simulink model "EMG_FES2_simulations"  (R2020b)
settings: Solver=FixedStepAuto  StartTime=0.0  StopTime=500  FixedStep=1/Fs  RelTol=1e-3  EnableMultiTasking=on
InitFcn:
  | Fs=1000;%Hz
undefined symbols (not defined in the file or in its folder): fdesignblkfcn, gcbh
libraries: simulink x3, dspswit3 x3, dspinverses x3, dspfdesign x1, dspstat3 x1
settings Model: Creator=bethel.osuagwu  LastModifiedBy=julie
settings DataIOCC: LimitDataPoints=on  SaveFormat=Array  ReturnWorkspaceOutputs=off
settings OptimizationCC: LifeSpan=inf
settings DebuggingCC: SolverPrmCheckMsg=warning  SFUnexpectedBacktrackingDiag=warning  SFNoUnconditionalDefaultTransitionDiag=warning  SFExecutionAtInitializationDiag=none  ArithmeticOperatorsInVariantConditions=warning
settings HardwareCC: ProdBitPerPointer=32  ProdBitPerSizeT=32  ProdBitPerPtrDiffT=32  ProdLargestAtomicFloat=None  ProdIntDivRoundTo=Undefined  ProdEndianess=Unspecified  ProdWordSize=32  ProdHWDeviceType=32-bit Generic
settings ModelReferenceCC: PropagateSignalLabelsOutOfModel=off
settings SFSimCC: SimUseLocalCustomCode=off  CustomCodeUndefinedFunction=UseInterfaceOnly
settings RTWCC: RTWUseLocalCustomCode=off
settings CodeAppCC: StateflowObjectComments=on
settings GRTTargetCC: TargetLangStandard=C89/C90 (ANSI)
settings ConfigComp: CovMetricSettings=dw  CovSaveCumulativeToWorkspaceVar=on  CovSaveSingleToWorkspaceVar=on  CovExternalEMLEnable=off  CovSFcnEnable=off

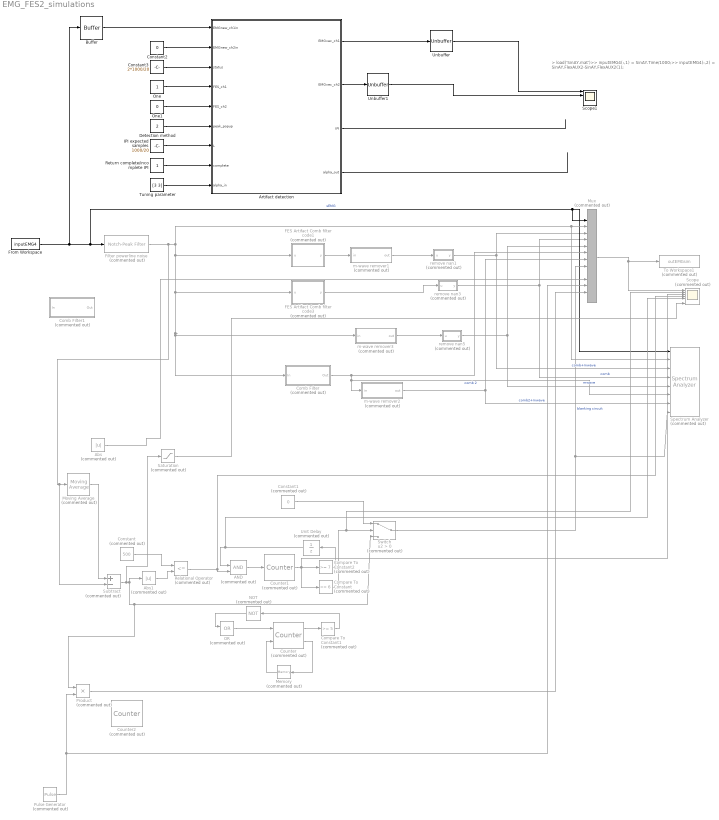
== system EMG_FES2_simulations ==
  note: > load('SinAY.mat')>> inputEMG4(:,1) = SinAY.Time/1000;>> inputEMG4(:,2) = SinAY.FlexAUX2-SinAY.FlexAUX2(1);
  AND : Logic  Commented=on  IconShape=distinctive  AllPortsSameDT=off  OutDataTypeStr=boolean
  Abs : Abs  Commented=on
  Abs1 : Abs  Commented=on
  Artifact detection : MATLAB Function  TreatAsAtomicUnit=on
  Buffer : Buffer  N=2*1000/20  OutputFrames=off
  Comb Filter : Subsystem  Commented=on  DialogController=fdesignblkfcn  InitFcn=fdesignblkfcn(gcbh, {'InitFcn'});  mask(Comb Filter){}
      mask help: Design a Comb Filter
      settings: CopyFcn=fdesignblkfcn(gcbh, {'CopyFcn'});
      mask Help: helpview(mapfilelocation('dsp'), 'dspcombfilter');
      mask Display: disp('Comb');
  Comb Filter1 : Subsystem  Commented=on  DialogController=fdesignblkfcn  InitFcn=fdesignblkfcn(gcbh, {'InitFcn'});  mask(Comb Filter){}
      mask help: Design a Comb Filter
      settings: CopyFcn=fdesignblkfcn(gcbh, {'CopyFcn'});
      mask Help: helpview(mapfilelocation('dsp'), 'dspcombfilter');
      mask Display: disp('Comb');
  Compare To Constant : simulink/Logic and Bit Operations/Compare To Constant  Commented=on  relop=<=  const=6  OutDataTypeStr=boolean
  Compare To Constant1 : simulink/Logic and Bit Operations/Compare To Constant  Commented=on  relop=>=  const=5  OutDataTypeStr=boolean
  Compare To Constant2 : simulink/Logic and Bit Operations/Compare To Constant  Commented=on  relop=>=  const=7  OutDataTypeStr=boolean
  Constant : Constant  Commented=on  Value=500
  Constant1 : Constant  Commented=on  Value=0
  Constant2 : Constant  Value=0
  Constant3 : Constant  Value=2*1000/20
  Counter : dspswit3/Counter  Commented=on  Direction=Up  CountEvent=Non-zero sample  CounterSize=User defined  MaxCount=5  InitialCount=0  Output=Count and Hit  HitValue=5  ResetInput=on  SamplesPerFrame=1  Ts=1  CntDtype=double  HitDtype=Logical
  Counter1 : dspswit3/Counter  Commented=on  Direction=Up  CountEvent=Free running  CounterSize=User defined  MaxCount=1000  InitialCount=0  Output=Count  HitValue=5  ResetInput=on  SamplesPerFrame=1  Ts=-1  CntDtype=double  HitDtype=Logical
  Counter2 : dspswit3/Counter  Commented=on  Direction=Up  CountEvent=Free running  CounterSize=User defined  MaxCount=255  InitialCount=0  Output=Count and Hit  HitValue=50  ResetInput=on  SamplesPerFrame=1  Ts=-1  CntDtype=double  HitDtype=Logical
  Detection method : Constant  Value=2
  FES Artifact Comb filter code1 : MATLAB Function  Commented=on  TreatAsAtomicUnit=on
  FES Artifact Comb filter code3 : MATLAB Function  Commented=on  TreatAsAtomicUnit=on
  Filter powerline noise : dspfdesign/Notch-Peak Filter  Commented=on  Specification=Quality factor and center frequency  BandwidthPort=off  Bandwidth=50  QualityFactorPort=off  QualityFactor=32  CenterFrequencyPort=off  CenterFrequency=50  BandwidthCoefficientPort=off  BandwidthCoefficient=0.72654  CenterFrequencyCoefficientPort=off  CenterFrequencyCoefficient=0  Output=Notch  InheritSampleRate=off  SampleRate=1000  SimulateUsing=Code generation
      settings: SourceProductBaseCode=DS
  From Workspace : FromWorkspace  VariableName=inputEMG4  SampleTime=1/Fs  OutputAfterFinalValue=Setting to zero
  IPI expected samples : Constant  Value=1000/20
  Memory : Memory  Commented=on
  Moving Average : dspstat3/Moving Average  Commented=on  Method=Sliding window  ForgettingFactorPort=off  SpecifyWindowLength=on  WindowLength=2000  ForgettingFactor=0.9  SimulateUsing=Code generation
  Mux : Mux  Commented=on  Inputs=12
  NOT : Logic  Commented=on  Operator=NOT  IconShape=distinctive  AllPortsSameDT=off  OutDataTypeStr=boolean
  OR : Logic  Commented=on  Operator=OR  IconShape=distinctive  AllPortsSameDT=off  OutDataTypeStr=boolean
  One : Constant  OutDataTypeStr=Inherit: Inherit via back propagation
  One1 : Constant  Value=0  OutDataTypeStr=Inherit: Inherit via back propagation
  Product : Product  Commented=on
  Pulse Generator : DiscretePulseGenerator  Commented=on  Period=50  PulseWidth=40  PhaseDelay=10  SampleTime=-1
  Relational Operator : RelationalOperator  Commented=on  Operator=<=  OutDataTypeStr=boolean  RndMeth=Simplest
  Return complete/incomplete IPI : Constant
  Saturation : Saturate  Commented=on  UpperLimit=250  LowerLimit=-250
  Scope : Scope  Commented=on  NumInputPorts=7
  Scope1 : Scope  NumInputPorts=4
  Spectrum Analyzer : SpectrumAnalyzer  Commented=on  NumInputPorts=8
  Subtract : Sum  Commented=on  Inputs=+-
  Switch : Switch  Commented=on  Criteria=u2 > Threshold
  To Workspace1 : ToWorkspace  Commented=on  VariableName=outEMGsim  SampleTime=-1
  Tuning parameter : Constant  Value=[3 3]
  Unbuffer : Unbuffer
  Unbuffer1 : Unbuffer
  Unit Delay : UnitDelay  Commented=on  SampleTime=-1  HasFrameUpgradeWarning=on
  m-wave remover1 : Subsystem  Commented=on
  m-wave remover2 : Subsystem  Commented=on
  m-wave remover3 : Subsystem  Commented=on
  remove nan1 : MATLAB Function  Commented=on  TreatAsAtomicUnit=on
  remove nan3 : MATLAB Function  Commented=on  TreatAsAtomicUnit=on
  remove nan5 : MATLAB Function  Commented=on  TreatAsAtomicUnit=on
  wires:
  Mux/1 -> To Workspace1/1, Scope/1
  m-wave remover3/1(out) -> remove nan5/1(u)
  FES Artifact Comb filter code3/1(y) -> remove nan3/1(u)
  m-wave remover1/1(out) -> remove nan1/1(u)
  FES Artifact Comb filter code1/1(y) -> m-wave remover1/1(in)
  remove nan1/1(y) -> Spectrum Analyzer/3, Mux/3  "comb+mwave"
  remove nan3/1(y) -> Spectrum Analyzer/4, Mux/4  "comb"
  remove nan5/1(y) -> Spectrum Analyzer/5, Mux/5  "mwave"
  From Workspace/1 -> Buffer/1, Filter powerline noise/1, Spectrum Analyzer/1, Mux/1  "sEMG"
  Filter powerline noise/1 -> Subtract/2, Moving Average/1, FES Artifact Comb filter code1/1(u), FES Artifact Comb filter code3/1(u), m-wave remover3/1(in), Comb Filter/1(In), Mux/2, Spectrum Analyzer/2
  Comb Filter/1(Out) -> m-wave remover2/1(in), Spectrum Analyzer/6, Mux/6  "comb 2"
  m-wave remover2/1(out) -> Spectrum Analyzer/7, Mux/7  "comb2+mwave"
  Switch/1 -> Spectrum Analyzer/8, Mux/8  "blanking circuit"
  Abs/1 -> Mux/10
  Moving Average/1 -> Subtract/1
  Constant/1 -> Relational Operator/1
  Subtract/1 -> Saturation/1, Abs1/1, Product/1, Switch/3
  Constant1/1 -> Switch/1
  Relational Operator/1 -> Scope/4, AND/2
  Memory/1 -> Counter/2
  NOT/1 -> OR/1
  OR/1 -> Counter/1
  Counter/2 -> Memory/1
  Compare To Constant1/1 -> NOT/1
  Counter/1 -> Compare To Constant1/1
  AND/1 -> Counter1/1
  Counter1/1 -> Compare To Constant/1, Scope/3, Compare To Constant2/1
  Compare To Constant/1 -> Scope/2, Switch/2
  Unit Delay/1 -> Scope/5, AND/1
  Compare To Constant2/1 -> Unit Delay/1
  Abs1/1 -> Relational Operator/2
  Saturation/1 -> Scope/7
  Pulse Generator/1 -> Mux/11, Product/2
  Product/1 -> Mux/12
  Detection method/1 -> Artifact detection/6(peak_popup)
  Tuning parameter/1 -> Artifact detection/9(alpha_in)
  IPI expected samples/1 -> Artifact detection/7(L)
  Return complete/incomplete IPI/1 -> Artifact detection/8(complete)
  One/1 -> Artifact detection/4(FES_ch1)
  One1/1 -> Artifact detection/5(FES_ch2)
  Constant2/1 -> Artifact detection/2(EMGnew_ch2in)
  Buffer/1 -> Artifact detection/1(EMGnew_ch1in)
  Constant3/1 -> Artifact detection/3(status)
  Artifact detection/2(EMGvec_ch2) -> Unbuffer1/1
  Artifact detection/1(EMGvec_ch1) -> Unbuffer/1
  Unbuffer/1 -> Scope1/1
  Unbuffer1/1 -> Scope1/2
  Artifact detection/3(IPI) -> ?
  Artifact detection/4(alpha_out) -> ?

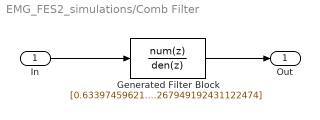
== system EMG_FES2_simulations/Comb Filter ==
  In : Inport
  Generated Filter Block : DiscreteFilter  Tag=BlockMethodSubSystem  Numerator=[0.633974596215561292 0 0 0 0 0 0 0 0 0 0 0 0 0 0 0 0 0 0 0 0 0 0 0 0 0 0 0 0 0 0 0 0 0 0 0 0 0 0 0 0 0 0 0 0 0 0 0 0 0 -0.633974596215561292]  Denominator=[1 0 0 0 0 0 0 0 0 0 0 0 0 0 0 0 0 0 0 0 0 0 0 0 0 0 0 0 0 0 0 0 0 0 0 0 0 0 0 0 0 0 0 0 0 0 0 0 0 0 -0.267949192431122474]  InputProcessing=Columns as channels (frame based)  FilterStructure=Direct form II transposed  a0EqualsOne=on
  Out : Outport  VectorParamsAs1DForOutWhenUnconnected=off
  wires:
  Generated Filter Block/1 -> Out/1
  In/1 -> Generated Filter Block/1

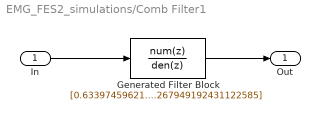
== system EMG_FES2_simulations/Comb Filter1 ==
  In : Inport
  Generated Filter Block : DiscreteFilter  Tag=BlockMethodSubSystem  Numerator=[0.633974596215561292 0 0 0 0 0 0 0 0 0 0 0 0 0 0 0 0 0 0 0 -0.633974596215561292]  Denominator=[1 0 0 0 0 0 0 0 0 0 0 0 0 0 0 0 0 0 0 0 -0.267949192431122585]  InputProcessing=Columns as channels (frame based)  a0EqualsOne=on
  Out : Outport  VectorParamsAs1DForOutWhenUnconnected=off
  wires:
  Generated Filter Block/1 -> Out/1
  In/1 -> Generated Filter Block/1

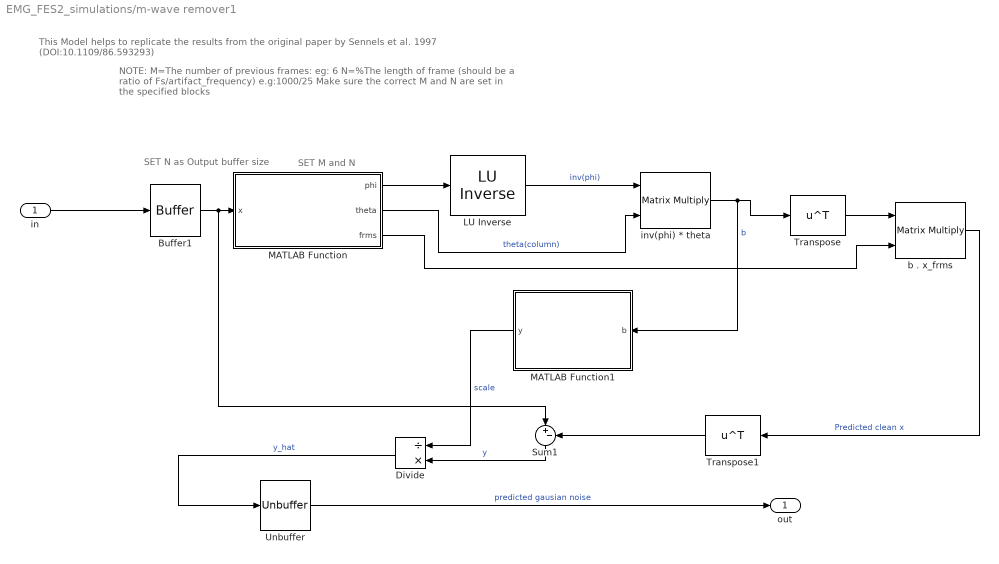
== system EMG_FES2_simulations/m-wave remover1 ==
  note: This Model helps to replicate the results from the original paper by Sennels et al. 1997 (DOI:10.1109/86.593293)
  note: SET M and N
  note: SET N as Output
      | buffer size
  note: NOTE:
      | M=The number of previous frames: eg: 6
      | N=%The length of frame (should be a ratio of Fs/artifact_frequency) e.g:1000/25
      | Make sure the correct M and N are set in the specified blocks
  in : Inport
  " LU Inverse" : dspinverses/ LU Inverse
  Buffer1 : Buffer  N=1000/20
  Divide : Product  Inputs=/*
  MATLAB Function : MATLAB Function  TreatAsAtomicUnit=on
  MATLAB Function1 : MATLAB Function  TreatAsAtomicUnit=on
  Sum1 : Sum  Inputs=|+-
  Transpose : Math  Operator=transpose  SaturateOnIntegerOverflow=on
  Transpose1 : Math  Operator=transpose  SaturateOnIntegerOverflow=on
  Unbuffer : Unbuffer
  b . x_frms : Product  Multiplication=Matrix(*)
  inv(phi) * theta : Product  Multiplication=Matrix(*)
  out : Outport
  wires:
  in/1 -> Buffer1/1
  Divide/1 -> Unbuffer/1  "y_hat"
  MATLAB Function1/1(y) -> Divide/1  "scale"
  Sum1/1 -> Divide/2  "y"
  Transpose1/1 -> Sum1/2
  b . x_frms/1 -> Transpose1/1  "Predicted clean x"
  Transpose/1 -> b . x_frms/1
  MATLAB Function/3(frms) -> b . x_frms/2
  Unbuffer/1 -> out/1  "predicted gausian noise"
  inv(phi) * theta/1 -> Transpose/1, MATLAB Function1/1(b)  "b"
  " LU Inverse"/1 -> inv(phi) * theta/1  "inv(phi)"
  MATLAB Function/2(theta) -> inv(phi) * theta/2  "theta(column)"
  MATLAB Function/1(phi) -> " LU Inverse"/1
  Buffer1/1 -> MATLAB Function/1(x), Sum1/1

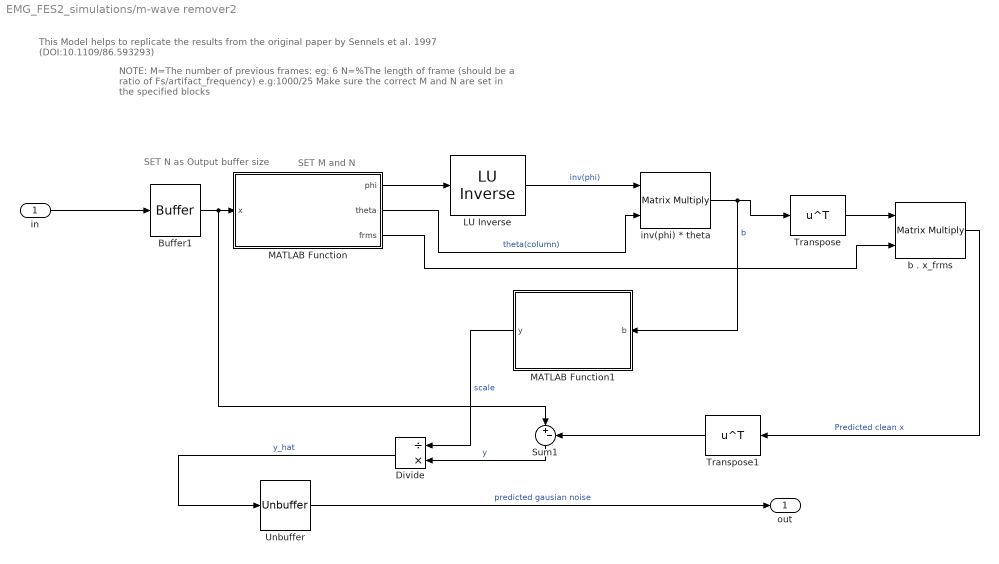
== system EMG_FES2_simulations/m-wave remover2 ==
  note: This Model helps to replicate the results from the original paper by Sennels et al. 1997 (DOI:10.1109/86.593293)
  note: SET M and N
  note: SET N as Output
      | buffer size
  note: NOTE:
      | M=The number of previous frames: eg: 6
      | N=%The length of frame (should be a ratio of Fs/artifact_frequency) e.g:1000/25
      | Make sure the correct M and N are set in the specified blocks
  in : Inport
  " LU Inverse" : dspinverses/ LU Inverse
  Buffer1 : Buffer  N=1000/20
  Divide : Product  Inputs=/*
  MATLAB Function : MATLAB Function  TreatAsAtomicUnit=on
  MATLAB Function1 : MATLAB Function  TreatAsAtomicUnit=on
  Sum1 : Sum  Inputs=|+-
  Transpose : Math  Operator=transpose  SaturateOnIntegerOverflow=on
  Transpose1 : Math  Operator=transpose  SaturateOnIntegerOverflow=on
  Unbuffer : Unbuffer
  b . x_frms : Product  Multiplication=Matrix(*)
  inv(phi) * theta : Product  Multiplication=Matrix(*)
  out : Outport
  wires:
  in/1 -> Buffer1/1
  Divide/1 -> Unbuffer/1  "y_hat"
  MATLAB Function1/1(y) -> Divide/1  "scale"
  Sum1/1 -> Divide/2  "y"
  Transpose1/1 -> Sum1/2
  b . x_frms/1 -> Transpose1/1  "Predicted clean x"
  Transpose/1 -> b . x_frms/1
  MATLAB Function/3(frms) -> b . x_frms/2
  Unbuffer/1 -> out/1  "predicted gausian noise"
  inv(phi) * theta/1 -> Transpose/1, MATLAB Function1/1(b)  "b"
  " LU Inverse"/1 -> inv(phi) * theta/1  "inv(phi)"
  MATLAB Function/2(theta) -> inv(phi) * theta/2  "theta(column)"
  MATLAB Function/1(phi) -> " LU Inverse"/1
  Buffer1/1 -> MATLAB Function/1(x), Sum1/1

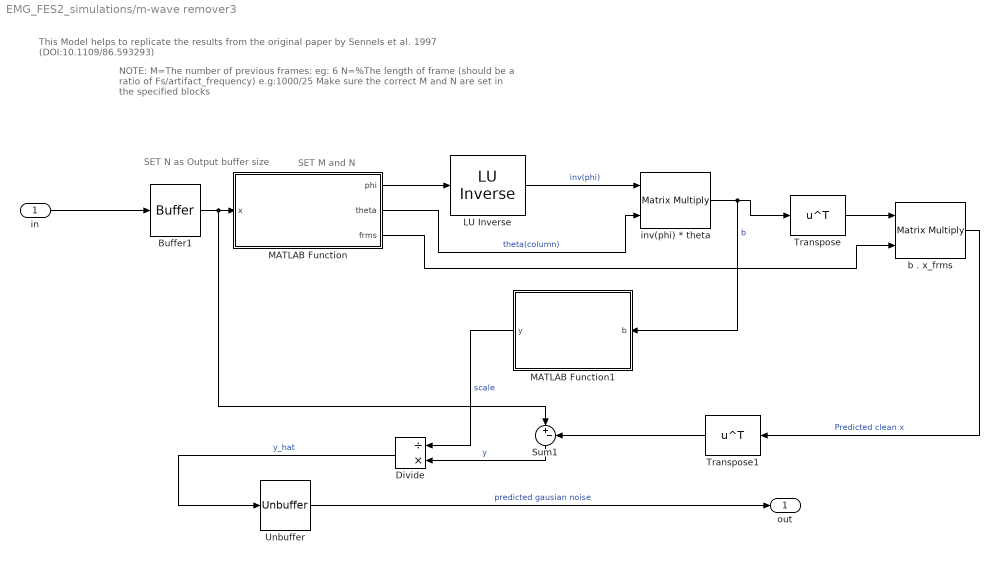
== system EMG_FES2_simulations/m-wave remover3 ==
  note: This Model helps to replicate the results from the original paper by Sennels et al. 1997 (DOI:10.1109/86.593293)
  note: SET M and N
  note: SET N as Output
      | buffer size
  note: NOTE:
      | M=The number of previous frames: eg: 6
      | N=%The length of frame (should be a ratio of Fs/artifact_frequency) e.g:1000/25
      | Make sure the correct M and N are set in the specified blocks
  in : Inport
  " LU Inverse" : dspinverses/ LU Inverse
  Buffer1 : Buffer  N=1000/20
  Divide : Product  Inputs=/*
  MATLAB Function : MATLAB Function  TreatAsAtomicUnit=on
  MATLAB Function1 : MATLAB Function  TreatAsAtomicUnit=on
  Sum1 : Sum  Inputs=|+-
  Transpose : Math  Operator=transpose  SaturateOnIntegerOverflow=on
  Transpose1 : Math  Operator=transpose  SaturateOnIntegerOverflow=on
  Unbuffer : Unbuffer
  b . x_frms : Product  Multiplication=Matrix(*)
  inv(phi) * theta : Product  Multiplication=Matrix(*)
  out : Outport
  wires:
  in/1 -> Buffer1/1
  Divide/1 -> Unbuffer/1  "y_hat"
  MATLAB Function1/1(y) -> Divide/1  "scale"
  Sum1/1 -> Divide/2  "y"
  Transpose1/1 -> Sum1/2
  b . x_frms/1 -> Transpose1/1  "Predicted clean x"
  Transpose/1 -> b . x_frms/1
  MATLAB Function/3(frms) -> b . x_frms/2
  Unbuffer/1 -> out/1  "predicted gausian noise"
  inv(phi) * theta/1 -> Transpose/1, MATLAB Function1/1(b)  "b"
  " LU Inverse"/1 -> inv(phi) * theta/1  "inv(phi)"
  MATLAB Function/2(theta) -> inv(phi) * theta/2  "theta(column)"
  MATLAB Function/1(phi) -> " LU Inverse"/1
  Buffer1/1 -> MATLAB Function/1(x), Sum1/1

== matlab function EMG_FES2_simulations/FES Artifact Comb filter code1 ==
  data: u input; y output
function y  = fcn(u)
%#codegen

persistent u_mem;
fes_freq=20;%FES frequency
Fs=1000;%EMG/data samplerate
K=round(Fs/fes_freq); %Comb filter order = (1/fes_freq)*Fs
a=-1;%{-1 to 0}
if isempty(u_mem)
    u_mem=zeros(K,1);
end





%% Comb filtering
% Forward comb
y=u+ a*u_mem(1);



u_mem(1:end-1)=u_mem(2:end);
u_mem(end)=u;
end





%

== matlab function EMG_FES2_simulations/FES Artifact Comb filter code3 ==
  data: u input; y output
function y  = fcn(u)
%#codegen

persistent u_mem;
fes_freq=20;%FES frequency
Fs=1000;%EMG/data samplerate
K=round(Fs/fes_freq); %Comb filter order = (1/fes_freq)*Fs
a=-1;%{-1 to 0}
if isempty(u_mem)
    u_mem=zeros(K,1);
end





%% Comb filtering
% Forward comb
y=u+ a*u_mem(1);



u_mem(1:end-1)=u_mem(2:end);
u_mem(end)=u;
end





%

== matlab function EMG_FES2_simulations/m-wave remover2/MATLAB Function ==
  data: x input; phi output double; theta output; frms output
function [phi,theta,frms] = fcn(x)
%#codegen
persistent t_sample phi_mem  frms_mem ;

%General param
M=6; %The number of previous frames 
N=1000/20; %The length of frame (should be a ratio of Fs/artifact_frequency)

% Performance parameter
freshPhi =1;% when =1:recompute phi(covariance matix) all the phi; when =0:update phi with only new values

if isempty(t_sample)
    t_sample=0;
    frms_mem=zeros(M,N);
    
    phi_mem=zeros(M,M);
end
t_sample=t_sample+1;

%make x a row vector
x=x';


%% compute phi
frms=frms_mem;
%equ 7 and 8
if(freshPhi)
    % compute phi fresh all the time
    phi=(frms*frms');
else
    %we can compute only the required column (first) and row (first)of phi
    %matrix and push the new values into phi
    phi_mem(2:end,2:end)=phi_mem(1:end-1,1:end-1);
    phi_mem(1,:)=frms(1,:)*frms';
    phi_mem(:,1)=phi_mem(1,:)';
    %phi-phi_mem
    phi=phi_mem;
end


%% compute theta
theta=(x*frms')';
%t_sample
%if t_sample==15
%    y=4;
%end


%% update frame
frms_mem(2:end,:)=frms_mem(1:end-1,:);
frms_mem(1,:)=x;

== matlab function EMG_FES2_simulations/remove nan1 ==
  data: u input; y output
function y  = fcn(u)
%#codegen

y=u;
if isnan(y)
    y=0;
end





%

== matlab function EMG_FES2_simulations/m-wave remover2/MATLAB Function1 ==
  data: b input; y output
function y = fcn(b)
%#codegen


y = sqrt(1+sum(b.^2));
%       OR
%y = (1+sum(b));%approximated for speed

== matlab function EMG_FES2_simulations/remove nan3 ==
  data: u input; y output
function y  = fcn(u)
%#codegen

y=u;
if isnan(y)
    y=0;
end





%

== matlab function EMG_FES2_simulations/Artifact detection ==
  data: EMGnew_ch1in input; EMGvec_ch1 output; EMGnew_ch2in input; status input; FES_ch1 input; FES_ch2 input; peak_popup input; L input; complete input; alpha_in input; EMGvec_ch2 output; IPI output; alpha_out output
%% %%%%%%%%%%%%%%%%%%%%%%%%%%%%%%%%%%%%%%%%%%%%%%%%%%%%%%%%%%%%%%%%%%%%%%%%
% block artifactDetection
% by Ana de Sousa (anacsousa@lara.unb.br)
% Last update: Feb-2018
%% %%%%%%%%%%%%%%%%%%%%%%%%%%%%%%%%%%%%%%%%%%%%%%%%%%%%%%%%%%%%%%%%%%%%%%%%

function [EMGvec_ch1, EMGvec_ch2, IPI, alpha_out]   = artifactDetection(EMGnew_ch1in, EMGnew_ch2in, status, FES_ch1, FES_ch2, peak_popup, L, complete, alpha_in)

    %% transpose if not column
    if isrow(EMGnew_ch1in)
        EMGnew_ch1 = EMGnew_ch1in';
    else
        EMGnew_ch1 = EMGnew_ch1in;
    end    
    if isrow(EMGnew_ch2in)
        EMGnew_ch2 = EMGnew_ch2in';
    else
        EMGnew_ch2 = EMGnew_ch2in;
    end

    %% Definition of parameters  
    b = 3.1;
    buffer_size = ceil(L*b);
    buffer_offsets_size = 5;
    n_stims = floor(b)+1;   
    ch_conn = [0,0];
    
    %% Step 0: pre-check (Verification of connected channels)
    if EMGnew_ch1 == 0
        ch_conn(1) = 0;
    else
        ch_conn(1) = 1;
    end
    
    if EMGnew_ch2 == 0
        ch_conn(2) = 0;
    else
        ch_conn(2) = 1;
    end
    
    %% Step 1: create and update buffers
    persistent  emg_buffer; 
    if isempty(emg_buffer)
        emg_buffer = bound_buffer2(buffer_size);
    end
    
    persistent  buffer_offsets_ch1;
    if isempty(buffer_offsets_ch1) 
        buffer_offsets_ch1 = bound_buffer(buffer_offsets_size);
    end
    
    persistent  buffer_offsets_ch2;
    if isempty(buffer_offsets_ch2) 
        buffer_offsets_ch2 = bound_buffer(buffer_offsets_size);
    end
    
    persistent  last_stim; 
    if isempty(last_stim)
        last_stim = bound_stim(n_stims);
    end
    
    %% alpha definitions
    persistent  alpha;
    if isempty(alpha) 
        alpha = alpha_in(2); % init alpha with second value
    end
    
    % Updates buffer from EMG data
    EMGstatus = int16(status(1));
    
    if (EMGstatus >= 1)   % ch1
        if EMGstatus > buffer_size % limit EMGstatus size to avoid errors if incorrect freq is put
            EMGstatus = int16(buffer_size);
            disp('Warning: status > buffer size, check EMG and stimulation frequencies.');
        end
        if size(EMGnew_ch1,1) > 1
            emg_buffer(1:buffer_size,1) = [emg_buffer(EMGstatus+1:buffer_size,1);EMGnew_ch1(1:EMGstatus)];
        end
    end
    
    if (EMGstatus >= 1)   % ch2
        if size(EMGnew_ch2,1) > 1
            emg_buffer(1:buffer_size,2) = [emg_buffer(EMGstatus+1:buffer_size,2);EMGnew_ch2(1:EMGstatus)];
        end
    end
    
    % Updates buffer from FES data
    stim = or(FES_ch1(1),FES_ch2(1));    
    last_stim(1:n_stims) = [last_stim(2:n_stims);stim];
    idx = last_stim ~= 0; 
    n_stims = sum(idx(:)); % # of artifacts expected, relates to buff_size;
        
    %% Step 2: artifacts detection (all artifacts found)
    IPI_c = buffer_size - L;
    IPI_i = buffer_size - L;
    
    % considers if channels are conn and stimulated 
    if (ch_conn(1)==1)||(ch_conn(2)==1) 
        if n_stims % if there is any pulse
            
            if (~isequal(last_stim,[0;0;0;1]))&&(~isequal(last_stim,[1;0;0;0])) % transitions of stim
                % find all points
                [all_pts] = choose_algorithm(peak_popup,alpha,emg_buffer);
                
                    %% consider # clusters vs alpha 
                    n_clusters = count_clusters(all_pts,L);
                    
                    %% if automatic alpha was chosen:
                    if alpha_in(1)
                        n_exp_pulses = 3;                        
                        d_alpha = n_clusters - n_exp_pulses;
                        
                        % if found pulses are different from expected pulses
                        if ~((n_clusters == 3) || (n_clusters == 4) || (n_clusters == 5))
                            % alpha limits
                            switch peak_popup
                                case 1 % 'var'
                                    ss = 0.1;
                                    alpha = alpha*(1+sign(d_alpha)*ss);
                                    
                                    if alpha < 10^-3
                                        alpha = 10^-3;
                                    elseif alpha > 5
                                        alpha = 5;
                                    end
                                    
                                case 2 % 'MAD'  
                                    ss = 0.1;
                                    alpha = alpha*(1+sign(d_alpha)*ss);
                                    
                                    if alpha < 2
                                        alpha = 2;
                                    elseif alpha > 5000
                                        alpha = 5000;
                                    end
                                case 3 % 'q'   
                                    ss = 0.01;
                                    alpha = alpha*(1+sign(d_alpha)*ss);
                                    
                                    if alpha < 0.9 %% simulink does not understand that we already bounded it...
                                        alpha = 0.9;
                                    elseif alpha >  0.985
                                        alpha = 0.985;
                                    end
                                otherwise % 'otherwise'
                                    error('No algorithm was selected.');
                            end   
                        end
                    end

                %% Step 3: determine IPI based on found artifacts
                [IPI_c,IPI_i] = cluster_peaks(all_pts, L, last_stim, n_stims);
            end
        end
    end
    
    %% Step 4: extract last full emg period
    if complete % return IPI complete or incomplete
        IPI = IPI_c;        
        % check if enough samples  
        if (IPI(1) < 0 )||(IPI(1) > buffer_size - L) 
            IPI(1) = buffer_size - L;
        end
    else
        IPI = IPI_i;
    end
    
    [ EMGvec_ch1, buffer_offsets_ch1 ] = extractLastFullEMG(IPI, emg_buffer(:,1), buffer_offsets_ch1, L, complete); 
    [ EMGvec_ch2, buffer_offsets_ch2 ] = extractLastFullEMG(IPI, emg_buffer(:,2), buffer_offsets_ch2, L, complete);
    
    alpha_out = alpha;
end

%% %%%%%%%%%%%%%%%%%%%%%%%%%%%%%%%%%%%%%%%%%%%%%%%%%%%%%%%%%%%%%%%%%%%%%%%%%
%% %%%%%%%%%%%%%%%%%%%%%%%%%%%%%%%%%%%%%%%%%%%%%%%%%%%%%%%%%%%%%%%%%%%%%%%%%
%% %%%%%%%%%%%%%%%%%%%%%%%%%%%%%%%%%%%%%%%%%%%%%%%%%%%%%%%%%%%%%%%%%%%%%%%%%

%% Specify Upper Bounds for Local Variables
% see more: (https://de.mathworks.com/help/simulink/ug/variable-size-data-when-dynamic-memory-allocation-is-disabled.html)
function y = bound_buffer(n)
    assert(n <= 5*4000/10, 'Buffer size is higher than 2000.'); 
    y = zeros(n,1);
end

function y = bound_buffer2(n)
    assert(n <= 5*4000/10, 'Buffer size is higher than 2000.');
    y = zeros(n,2);
end

function y = bound_stim(n)
    assert(n <= 10, 'Number of stims is higher than 10. '); 
    y = zeros(n,1);
end

function y = bound_vec(n)
    assert(n <= 5*4000/10, 'Buffer size is higher than 2000.'); 
    y = zeros(1,n);
end

%% Choose the algorithm to find all peaks %%%%%%%%%%%%%%%%%%%%%%%%%%%%%%%%%
function [all_IPI] = choose_algorithm(peak_popup,alpha,emg_vec)
    n_loc_found = length(emg_vec);
    all_IPI = zeros(1,n_loc_found);
    
    switch peak_popup
        case 1 % 'std'            
            DE1 = (diff(diff(emg_vec(:,1))));
            DE2 = (diff(diff(emg_vec(:,2))));
            mean_d1 = mean(DE1,'omitnan');  mean_d2 = mean(DE2,'omitnan');
            std_d1 = std(DE1,'omitnan');    std_d2 = std(DE2,'omitnan');
            
            % look for points
            k_max1 = mean_d1+std_d1*alpha;  k_max2 = mean_d2+std_d2*alpha;
            k_min1 = mean_d1-std_d1*alpha;  k_min2 = mean_d2-std_d2*alpha;
            
            loc_found1 = find(DE1 > k_max1 | DE1 < k_min1); %find std1
            loc_found2 = find(DE2 > k_max2 | DE2 < k_min2); %find std2
            loc_found = union(loc_found1,loc_found2);

        case 2 % 'MAD'
            DE1 = (diff(diff(emg_vec(:,1))));
            DE2 = (diff(diff(emg_vec(:,2))));
            mean_d1 = median(DE1,'omitnan');  mean_d2 = median(DE2,'omitnan');
            mad_d1 = mad(DE1,1);            mad_d2 = mad(DE2,1);
            
            % look for points
            k_max1 = mean_d1+mad_d1*alpha;  k_max2 = mean_d2+mad_d2*alpha;
            k_min1 = mean_d1-mad_d1*alpha;  k_min2 = mean_d2-mad_d2*alpha;
            
            loc_found1 = find(DE1 > k_max1 | DE1 < k_min1); %find std1
            loc_found2 = find(DE2 > k_max2 | DE2 < k_min2); %find std2
            loc_found = union(loc_found1,loc_found2);
            
        case 3 % 'quantiles'
            DE1 = (diff(diff(emg_vec(:,1))));
            DE2 = (diff(diff(emg_vec(:,2))));
            
            
            if alpha < 0.9 %% simulink does not understand that we already bounded it...
                alpha = 0.9;
            elseif alpha >  0.985
                alpha = 0.985;
            end

            q_max1 = quantile(DE1,alpha);
            q_min1 = quantile(DE1,1-alpha);
            q_max2 = quantile(DE2,alpha); 
            q_min2 = quantile(DE2,1-alpha);
            loc_found1 = find( DE1>q_max1(1) | DE1<q_min1(1)) ; %find quantiles DE1
            loc_found2 = find( DE2>q_max2(1) | DE2<q_min2(1)) ; %find quantiles DE2
            loc_found = union(loc_found1,loc_found2);   
            
        otherwise % 'otherwise'
            error('No algorithm was selected.');
    end
    
    % Adjust vector to return
    if ~isempty(loc_found)
        a = min(n_loc_found,length(loc_found));  %check which is smaller

        for i=1:a % do not extrapolate the vector
            all_IPI(i) = loc_found(i);
        end
    end  
end

%% Extract last full emg period from last IPI %%%%%%%%%%%%%%%%%%%%%%%%%%%%%
function [ EMGvec, offsets_buffer ] = extractLastFullEMG(IPI, emg_buffer, offsets_buffer, L, complete)

	% Parameters
%     EMGvec = NaN(1,200);
    EMGvec = NaN(1,100);
    buffer_size = length(emg_buffer);
    buffer_size_offsets = length(offsets_buffer); 
    
    %% update the emg vec with the new COMPLETE peak (until L)
    
    %% if IPI is not zero, we return position based on IPI (complete or incomplete)
    if IPI(1) ~= 0
        %% now we consider if it is complete or incomplete
        if complete %% complete
            for i = 1:L 
                EMGvec(i) = emg_buffer(IPI + i);
            end
        else %% incomplete
            %% if there is enough samples, just fill (buffer_size-L)
            if IPI(1) <= buffer_size - L
                for i = 1:L 
                    EMGvec(i) = emg_buffer(IPI + i);
                end
            %% if there is not, fill until possible (buffer_size-IPI)
            else
                for i = 1:buffer_size-IPI 
                    EMGvec(i) = emg_buffer(IPI + i);
                end
            end
        end
    %% otherwise, something went wrong before, so return EMGvec as zero
    else
        for i = 1:L 
            EMGvec(i) = 0;
        end
    end
        
    %% Remove offset
    for i = 1:buffer_size_offsets-1
        offsets_buffer(end-i+1) = offsets_buffer(end-i);
    end
    x = 0;
    c = buffer_size_offsets;
    for i = 1:buffer_size_offsets
        x = x + emg_buffer(ceil(0.8*L) + i);
    end
    offsets_buffer(1) = x/c; %mean

    EMGvec = EMGvec - mean(offsets_buffer);
    EMGvec = EMGvec.'; % return
end


%% Cluster peaks %%%%%%%%%%%%%%%%%%%%%%%%%%%%%%%%%%%%%%%%%%%%%%%%%%%%%%%%%%%
function [IPI_c,IPI_i] = cluster_peaks(all_pts, L, last_stim, n_stims)

    %% parameters
    buffer_size = length(all_pts);
    if ~(last_stim(end) == 0) %adjust # of expected stims
        n_stims = n_stims-1;
    end
    
    %% find clusters and count # of elements in each cluster
    ind_del = all_pts == 0;    points = all_pts;
    points(ind_del) = [];
    changes = find((diff(points) > L*0.1))+1; % find where cluster change
    n_clusters = length(changes) + 1; % # of clusters found
    
    a = zeros(1,n_clusters);
    b = zeros(1,n_clusters);
    
    if(n_clusters > 1) % more than one cluster found
        u = [changes(1)-1, diff(changes), length(points) - changes(end) + 1];        
        % saving first (a) and last (b) points of each cluster (i)
        for i=1:n_clusters
            if i == 1
                a(i) = points(1);
                b(i) = points(changes(i)-1);
            elseif i == n_clusters
                a(i) = points(changes(i-1));
                b(i) = points(end);
            else
                a(i) = points(changes(i-1));
                b(i) = points(changes(i)-1);
            end
        end
    else % only one (or none) cluster found
        u = length(points);
        if ~isempty(points)
            a = points(1);
            b = points(end);
        else
            a = 1;
            b = 1;
        end
    end
        
    %% create base and real vectors
    vec_base = bound_vec(buffer_size);    
    vec_real = bound_vec(buffer_size);
    
    if floor(mean(u)) % base
        if mean(b-a)+1 < ceil(L/2) % limit number of points
            n_pts = ceil(mean(b-a)+1);
        else
            n_pts = ceil(L/2);
        end
    else 
        n_pts = 5;
    end
    
    init = 1;    
    for i = 1:n_stims %vec_base
        vec_base((init + (i-1)*L):init + n_pts + (i-1)*L - 1) = 1;
    end
    
    for i = 1:length(a) %vec_real
        vec_real(a(i)) = 1;
        for j = 1:b(i)-a(i)
            vec_real(a(i)+j) = 1;
        end
    end
    
    %% Correlate vec_base and vec_real to shift them
    [acor,lag] = xcorr(vec_base', vec_real');
    [~,I] = max(abs(acor));
    lagDiff = abs(lag(I));
            
    %% Transition state (#stims = 1), IPI = lagDiff
    % Everthing bellow considers the transitions between on and off stim:
    %   . When the charge shifts on -> off, or off -> on, the stimulator
    %   needs a period to respond in real time.
    %   . Also we need to consider if we want a complete or an incomplete
    %   IPI.
    IPI_c = buffer_size - L;
    IPI_i = buffer_size - L;
    
    % TRANSITIONS
    adjust_diff = 0;
    if isequal(last_stim,[0;0;1;1]) % transition off->on (for IPI_i)
        IPI_i = lagDiff+adjust_diff;
        IPI_c = 0;
    elseif isequal(last_stim,[1;1;0;0]) % transition on->off (for IPI_c)
        new_pos = find( points > 0.95*(lagDiff+L+adjust_diff) ); % look for the 1st pulse after
        if new_pos
            IPI_c = points(new_pos(1))+adjust_diff;
        end
    elseif isequal(last_stim,[0;1;1;1]) % transition off->on (for in and complete)
        IPI_c = lagDiff+2;
        new_pos = find( points > 0.95*(lagDiff+L+adjust_diff) ); % look for next pulse
        if new_pos
            IPI_i = points(new_pos(1))+adjust_diff;
        end
    % STABLE
    else  
        new_pos = find( points > 0.95*(lagDiff+L+adjust_diff) ); % look for the 1st pulse after
        if new_pos
            IPI_c = points(new_pos(1))+adjust_diff;
        end

        new_pos2 = find( points > 0.95*(lagDiff+2*L+adjust_diff) ); % look for the 2nd pulse after
        if new_pos2
            IPI_i = points(new_pos2(1))+adjust_diff;
        end
    end
end

%% Count number of clusters %%%%%%%%%%%%%%%%%%%%%%%%%%%%%%%%%%%%%%%%%%%%%%%%
function n_clusters = count_clusters(all_pts,L)
    % make a vector without the zeros
    ind_del = all_pts == 0;     points = all_pts;
    points(ind_del) = [];  
    
    % count clusters considering a min diff between points
    changes = find((diff(points) > L*0.1))+1;
    n_clusters = length(changes) + 1;
end

== matlab function EMG_FES2_simulations/remove nan5 ==
  data: u input; y output
function y  = fcn(u)
%#codegen

y=u;
if isnan(y)
    y=0;
end





%

== matlab function EMG_FES2_simulations/m-wave remover1/MATLAB Function ==
  data: x input; phi output double; theta output; frms output
function [phi,theta,frms] = fcn(x)
%#codegen
persistent t_sample phi_mem  frms_mem ;

%General param
M=6; %The number of previous frames 
N=1000/20; %The length of frame (should be a ratio of Fs/artifact_frequency)

% Performance parameter
freshPhi =1;% when =1:recompute phi(covariance matix) all the phi; when =0:update phi with only new values

if isempty(t_sample)
    t_sample=0;
    frms_mem=zeros(M,N);
    
    phi_mem=zeros(M,M);
end
t_sample=t_sample+1;

%make x a row vector
x=x';


%% compute phi
frms=frms_mem;
%equ 7 and 8
if(freshPhi)
    % compute phi fresh all the time
    phi=(frms*frms');
else
    %we can compute only the required column (first) and row (first)of phi
    %matrix and push the new values into phi
    phi_mem(2:end,2:end)=phi_mem(1:end-1,1:end-1);
    phi_mem(1,:)=frms(1,:)*frms';
    phi_mem(:,1)=phi_mem(1,:)';
    %phi-phi_mem
    phi=phi_mem;
end


%% compute theta
theta=(x*frms')';
%t_sample
%if t_sample==15
%    y=4;
%end


%% update frame
frms_mem(2:end,:)=frms_mem(1:end-1,:);
frms_mem(1,:)=x;

== matlab function EMG_FES2_simulations/m-wave remover1/MATLAB Function1 ==
  data: b input; y output
function y = fcn(b)
%#codegen


y = sqrt(1+sum(b.^2));
%       OR
%y = (1+sum(b));%approximated for speed

== matlab function EMG_FES2_simulations/m-wave remover3/MATLAB Function ==
  data: x input; phi output double; theta output; frms output
function [phi,theta,frms] = fcn(x)
%#codegen
persistent t_sample phi_mem  frms_mem ;

%General param
M=6; %The number of previous frames 
N=1000/20; %The length of frame (should be a ratio of Fs/artifact_frequency)

% Performance parameter
freshPhi =1;% when =1:recompute phi(covariance matix) all the phi; when =0:update phi with only new values

if isempty(t_sample)
    t_sample=0;
    frms_mem=zeros(M,N);
    
    phi_mem=zeros(M,M);
end
t_sample=t_sample+1;

%make x a row vector
x=x';


%% compute phi
frms=frms_mem;
%equ 7 and 8
if(freshPhi)
    % compute phi fresh all the time
    phi=(frms*frms');
else
    %we can compute only the required column (first) and row (first)of phi
    %matrix and push the new values into phi
    phi_mem(2:end,2:end)=phi_mem(1:end-1,1:end-1);
    phi_mem(1,:)=frms(1,:)*frms';
    phi_mem(:,1)=phi_mem(1,:)';
    %phi-phi_mem
    phi=phi_mem;
end


%% compute theta
theta=(x*frms')';
%t_sample
%if t_sample==15
%    y=4;
%end


%% update frame
frms_mem(2:end,:)=frms_mem(1:end-1,:);
frms_mem(1,:)=x;

== matlab function EMG_FES2_simulations/m-wave remover3/MATLAB Function1 ==
  data: b input; y output
function y = fcn(b)
%#codegen


y = sqrt(1+sum(b.^2));
%       OR
%y = (1+sum(b));%approximated for speed
